simulink model "Fig06"  (R2023b)
settings: Solver=ode1  StartTime=0.0  StopTime=600  RelTol=1e-3
settings Model: Creator=orlandojorquera  LastModifiedBy=evogel

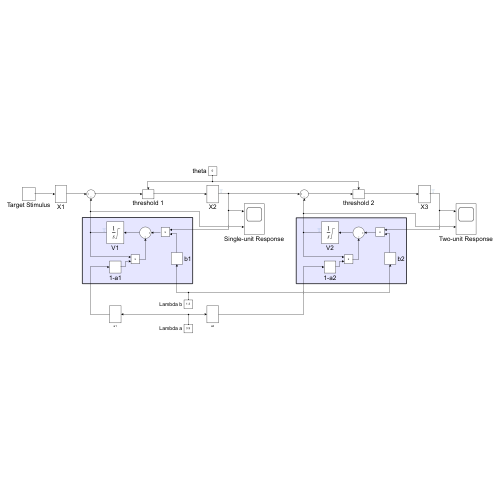
[thumbnail: Simulink's stored preview of the top-level diagram]
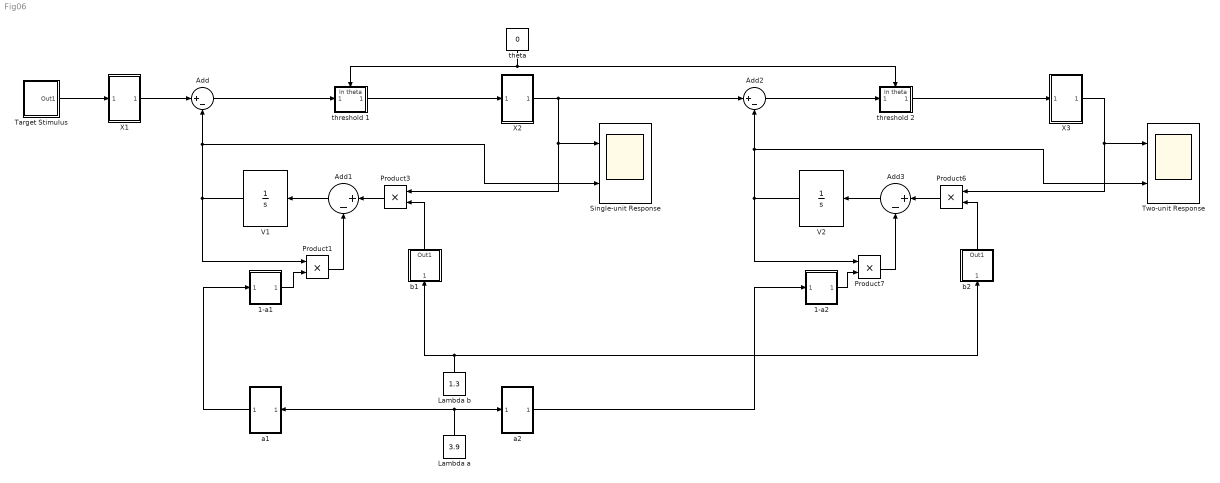
== system Fig06 ==
  1-a1 : Subsystem
  1-a2 : Subsystem
  Add{,1..3} (4 alike) : Sum  Inputs=|+-
  Lambda a : Constant  Value=3.9
  Lambda b : Constant  Value=1.3
  Product{1,3,6..7} (4 alike) : Product
  Single-unit Response : Scope  NumInputPorts=2
  Target Stimulus : Subsystem
  Two-unit Response : Scope  NumInputPorts=2
  V1 : Integrator  LimitOutput=on
  V2 : Integrator  LimitOutput=on
  X1 : Subsystem
  X2 : Subsystem
  X3 : Subsystem
  a1 : Subsystem
  a2 : Subsystem
  b1 : Subsystem
  b2 : Subsystem
  theta : Constant  Value=0
  threshold 1 : Subsystem
      settings: PortSchema="{\"entries\":[{\"content\":{\"sides\":[{\"content\":{\"connectorIds\":[\"In1\"]},\"type\":\"ConnectorPlacement.EquallySpacedRectSide\",\"uuid\":\"df45c11a-cbfd-46b0-9931-ccf6bdc824b5\"},{\"content\":{\"connectorIds\":[\"Out1\"],\"side\":\"RIGHT\"},\"type\":\"ConnectorPlacement.EquallySpacedRectSide\",\"uuid\":\"7bdc14d3-84cb-4ad0-a730-e3b8f98cb716\"},{\"content\":{\"connectorIds\":[\"In2\"],\"side\":\"TOP\"},\"type\":\"ConnectorPlacement.EquallySpacedRectSide\",\"uuid\":\"6aa308ce-d9e8-4768-ab82-80fe1eba77b8\"}]},\"type\":\"ConnectorPlacement.EquallySpacedConnector\",\"uuid\":\"5c730a05-bfd2-4eaa-b46f-f4851af60a3b\"}],\"packageUris\":[\"http://schema.mathworks.com/mf0/Connector/R2020b\"],\"version\":\"1.0\"}"
  threshold 2 : Subsystem
      settings: PortSchema="{\"entries\":[{\"content\":{\"sides\":[{\"content\":{\"connectorIds\":[\"In1\"]},\"type\":\"ConnectorPlacement.EquallySpacedRectSide\",\"uuid\":\"df45c11a-cbfd-46b0-9931-ccf6bdc824b5\"},{\"content\":{\"connectorIds\":[\"Out1\"],\"side\":\"RIGHT\"},\"type\":\"ConnectorPlacement.EquallySpacedRectSide\",\"uuid\":\"7bdc14d3-84cb-4ad0-a730-e3b8f98cb716\"},{\"content\":{\"connectorIds\":[\"In2\"],\"side\":\"TOP\"},\"type\":\"ConnectorPlacement.EquallySpacedRectSide\",\"uuid\":\"6aa308ce-d9e8-4768-ab82-80fe1eba77b8\"}]},\"type\":\"ConnectorPlacement.EquallySpacedConnector\",\"uuid\":\"5c730a05-bfd2-4eaa-b46f-f4851af60a3b\"}],\"packageUris\":[\"http://schema.mathworks.com/mf0/Connector/R2020b\"],\"version\":\"1.0\"}"
  wires:
  Target Stimulus/1(Out1) -> X1/1(In Stimulus)
  Lambda a/1 -> a1/1(In lambda_a), a2/1(In lambda_a)
  X1/1(Output) -> Add/1
  Add/1 -> threshold 1/1(In X1 - V1)
  theta/1 -> threshold 1/2(In theta), threshold 2/2(In theta)
  threshold 1/1(Out1) -> X2/1(In1)
  b1/1(Out1) -> Product3/2
  Product3/1 -> Add1/1
  Lambda b/1 -> b1/1(In lambda_b), b2/1(In lambda_b)
  Add1/1 -> V1/1
  V1/1 -> Product1/1, Add/2, Single-unit Response/2
  Product1/1 -> Add1/2
  Product7/1 -> Add3/2
  V2/1 -> Two-unit Response/2, Add2/2, Product7/1
  Add3/1 -> V2/1
  Product6/1 -> Add3/1
  b2/1(Out1) -> Product6/2
  threshold 2/1(Out1) -> X3/1(In1)
  Add2/1 -> threshold 2/1(In X2 - V2)
  a1/1(Out1) -> 1-a1/1(In a1)
  X2/1(Out1) -> Product3/1, Single-unit Response/1, Add2/1
  X3/1(Out1) -> Product6/1, Two-unit Response/1
  1-a1/1(Out1) -> Product1/2
  1-a2/1(Out1) -> Product7/2
  a2/1(Out1) -> 1-a2/1(In a2)

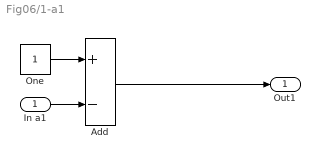
== system Fig06/1-a1 ==
  In a1 : Inport
  Add : Sum  Inputs=+-
  One : Constant  OutDataTypeStr=Inherit: Inherit via back propagation
  Out1 : Outport
  wires:
  One/1 -> Add/1
  Add/1 -> Out1/1
  In a1/1 -> Add/2

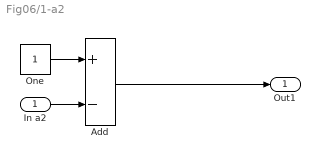
== system Fig06/1-a2 ==
  In a2 : Inport
  Add : Sum  Inputs=+-
  One : Constant  OutDataTypeStr=Inherit: Inherit via back propagation
  Out1 : Outport
  wires:
  In a2/1 -> Add/2
  Add/1 -> Out1/1
  One/1 -> Add/1

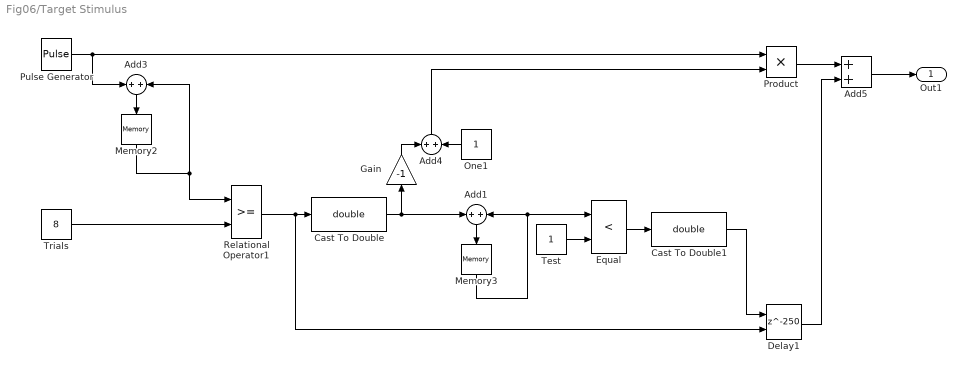
== system Fig06/Target Stimulus ==
  Add{1,3..5} (4 alike) : Sum
  Cast To Double : DataTypeConversion  OutDataTypeStr=double  SaturateOnIntegerOverflow=off  RndMeth=Floor
  Cast To Double1 : DataTypeConversion  OutDataTypeStr=double  SaturateOnIntegerOverflow=off  RndMeth=Floor
  Delay1 : Delay  DelayLength=250  ShowEnablePort=on
      settings: InputPortMap=u0,e6
  Equal : RelationalOperator  Operator=<  OutDataTypeStr=boolean  RndMeth=Simplest  InputSameDT=off
  Gain : Gain  Gain=-1
  Memory2 : Memory
  Memory3 : Memory
  One1 : Constant  OutDataTypeStr=Inherit: Inherit via back propagation
  Product : Product
  Pulse Generator : DiscretePulseGenerator  Period=10  PhaseDelay=180
  Relational Operator1 : RelationalOperator  OutDataTypeStr=boolean  RndMeth=Simplest  InputSameDT=off
  Test : Constant  OutDataTypeStr=Inherit: Inherit via back propagation
  Trials : Constant  Value=8
  Out1 : Outport
  wires:
  Pulse Generator/1 -> Add3/1, Product/1
  Add3/1 -> Memory2/1
  Memory2/1 -> Relational Operator1/1, Add3/2
  Trials/1 -> Relational Operator1/2
  Relational Operator1/1 -> Delay1/2, Cast To Double/1
  Cast To Double/1 -> Gain/1, Add1/1
  Add1/1 -> Memory3/1
  Memory3/1 -> Add1/2, Equal/1
  Test/1 -> Equal/2
  Equal/1 -> Cast To Double1/1
  Gain/1 -> Add4/1
  One1/1 -> Add4/2
  Add4/1 -> Product/2
  Cast To Double1/1 -> Delay1/1
  Product/1 -> Add5/1
  Delay1/1 -> Add5/2
  Add5/1 -> Out1/1

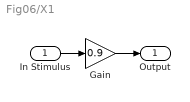
== system Fig06/X1 ==
  In Stimulus : Inport
  Gain : Gain  Gain=0.9
  Output : Outport
  wires:
  In Stimulus/1 -> Gain/1
  Gain/1 -> Output/1

== system Fig06/X2 ==
  In1 : Inport
  Out1 : Outport
  wires:
  In1/1 -> Out1/1

== system Fig06/X3 ==
  In1 : Inport
  Out1 : Outport
  wires:
  In1/1 -> Out1/1

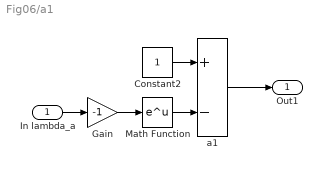
== system Fig06/a1 ==
  In lambda_a : Inport
  Constant2 : Constant
  Gain : Gain  Gain=-1
  Math Function : Math
  a1 : Sum  Inputs=+-
  Out1 : Outport
  wires:
  Math Function/1 -> a1/2
  Gain/1 -> Math Function/1
  Constant2/1 -> a1/1
  In lambda_a/1 -> Gain/1
  a1/1 -> Out1/1

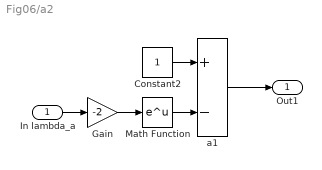
== system Fig06/a2 ==
  In lambda_a : Inport
  Constant2 : Constant
  Gain : Gain  Gain=-2
  Math Function : Math
  a1 : Sum  Inputs=+-
  Out1 : Outport
  wires:
  a1/1 -> Out1/1
  In lambda_a/1 -> Gain/1
  Constant2/1 -> a1/1
  Gain/1 -> Math Function/1
  Math Function/1 -> a1/2

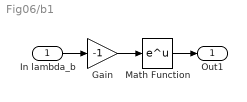
== system Fig06/b1 ==
  In lambda_b : Inport
  Gain : Gain  Gain=-1
  Math Function : Math
  Out1 : Outport
  wires:
  Math Function/1 -> Out1/1
  In lambda_b/1 -> Gain/1
  Gain/1 -> Math Function/1

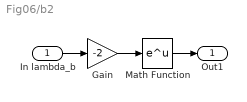
== system Fig06/b2 ==
  In lambda_b : Inport
  Gain : Gain  Gain=-2
  Math Function : Math
  Out1 : Outport
  wires:
  Gain/1 -> Math Function/1
  In lambda_b/1 -> Gain/1
  Math Function/1 -> Out1/1

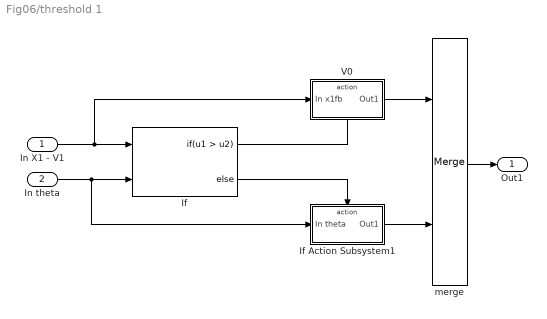
== system Fig06/threshold 1 ==
  In X1 - V1 : Inport
  In theta : Inport  Port=2
  If : If  NumInputs=2  IfExpression=u1 > u2
  If Action Subsystem1 : Subsystem  TreatAsAtomicUnit=on
  V0 : Subsystem  TreatAsAtomicUnit=on
  merge : Merge
  Out1 : Outport
  wires:
  V0/1(Out1) -> merge/1
  merge/1 -> Out1/1
  If Action Subsystem1/1(Out1) -> merge/2
  In theta/1 -> If Action Subsystem1/1(In theta), If/2
  In X1 - V1/1 -> V0/1(In x1fb), If/1
  If/1 -> V0/Action
  If/2 -> If Action Subsystem1/Action

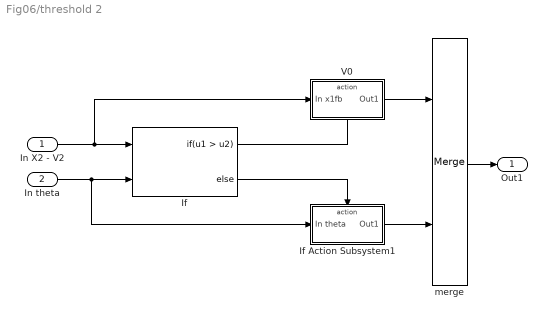
== system Fig06/threshold 2 ==
  In X2 - V2 : Inport
  In theta : Inport  Port=2
  If : If  NumInputs=2  IfExpression=u1 > u2
  If Action Subsystem1 : Subsystem  TreatAsAtomicUnit=on
  V0 : Subsystem  TreatAsAtomicUnit=on
  merge : Merge
  Out1 : Outport
  wires:
  If/2 -> If Action Subsystem1/Action
  If/1 -> V0/Action
  In X2 - V2/1 -> If/1, V0/1(In x1fb)
  In theta/1 -> If/2, If Action Subsystem1/1(In theta)
  If Action Subsystem1/1(Out1) -> merge/2
  merge/1 -> Out1/1
  V0/1(Out1) -> merge/1

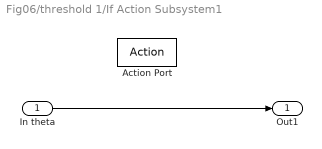
== system Fig06/threshold 1/If Action Subsystem1 ==
  In theta : Inport
  Action Port : ActionPort  ActionPortLabel=else
  Out1 : Outport
  wires:
  In theta/1 -> Out1/1

== system Fig06/threshold 1/V0 ==
  In x1fb : Inport
  Action Port : ActionPort  ActionPortLabel=if(u1 > u2)
  Out1 : Outport
  wires:
  In x1fb/1 -> Out1/1

== system Fig06/threshold 2/If Action Subsystem1 ==
  In theta : Inport
  Action Port : ActionPort  ActionPortLabel=else
  Out1 : Outport
  wires:
  In theta/1 -> Out1/1

== system Fig06/threshold 2/V0 ==
  In x1fb : Inport
  Action Port : ActionPort  ActionPortLabel=if(u1 > u2)
  Out1 : Outport
  wires:
  In x1fb/1 -> Out1/1
